simulink model "quad_with_controller"  (R2024b)
settings: configuration reference "prj_default_config" (kept outside this file)
values from neighbouring files (symbols this model uses):
  AngleRope_x = deg2rad(0)    [plant_init.m]
  AngleRope_z = deg2rad(0)    [plant_init.m]
  F_rope = 0    [plant_init.m]
  ModelInit_Att_p = 0    [plant_init.m]
  ModelInit_Att_phi = 0    [plant_init.m]
  ModelInit_Att_psi = 0    [plant_init.m]
  ModelInit_Att_q = 0    [plant_init.m]
  ModelInit_Att_r = 0    [plant_init.m]
  ModelInit_Att_theta = 0    [plant_init.m]
  ModelInit_Pos_Vx = 0    [plant_init.m]
  ModelInit_Pos_Vy = 0    [plant_init.m]
  ModelInit_Pos_Vz = 0    [plant_init.m]
  ModelInit_Pos_x = 0    [plant_init.m]
  ModelInit_Pos_y = 0    [plant_init.m]
  ModelInit_Pos_z = 0    [plant_init.m]
  ModelParam_c_M = 1.489e-07    [plant_init.m]
  ModelParam_c_T = 1.105e-05    [plant_init.m]
  ModelParam_d = 0.225    [plant_init.m]
  ModelParam_g = 9.8    [plant_init.m]
  ModelParam_I_xx = 1.314e-02    (= 0.01314)    [plant_init.m]
  ModelParam_I_yy = 1.314e-02    (= 0.01314)    [plant_init.m]
  ModelParam_I_zz = 2.375e-02    (= 0.02375)    [plant_init.m]
  ModelParam_J_RP = 0.0000986    (= 9.86e-05)    [plant_init.m]
  ModelParam_m = 1.5    [plant_init.m]
libraries: slpidlib x6, mqlib x2
settings Model: Creator=yangyu  LastModifiedBy=yangyu
settings ConfigSetRef: SourceName=prj_default_config  SourceLocation=Base Workspace

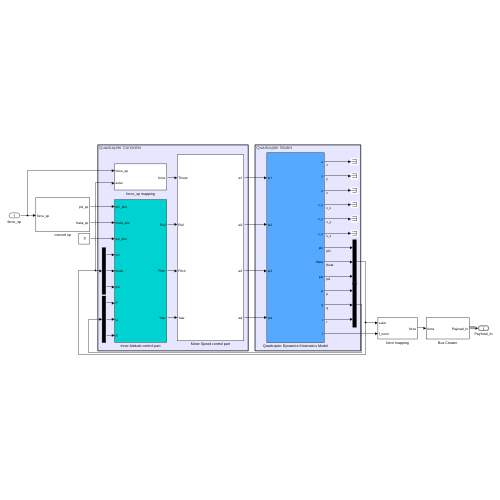
[thumbnail: Simulink's stored preview of the top-level diagram]
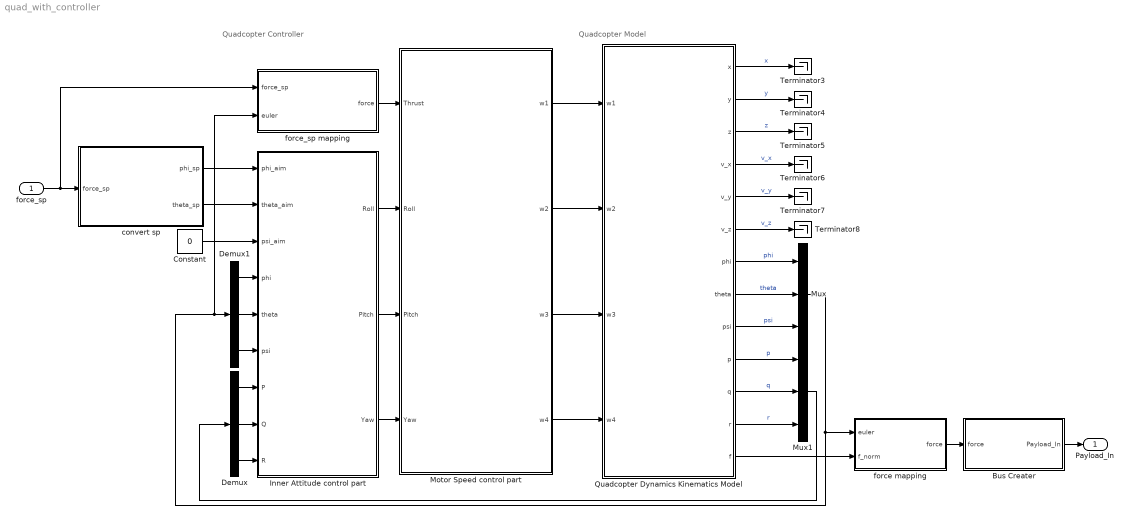
== system quad_with_controller ==
  note: Quadcopter Controller
  note: Quadcopter Model
  force_sp : Inport
  Bus Creater : Subsystem
  Constant : Constant  Value=0
  Demux : Demux  Outputs=3
  Demux1 : Demux  Outputs=3
  Inner Attitude control part : Subsystem
  Motor Speed control part : Subsystem
  Mux : Mux  Inputs=3
  Mux1 : Mux  Inputs=3
  Quadcopter Dynamics Kinematics Model : Subsystem
  Terminator{3..8} (6 alike) : Terminator
  convert sp : Subsystem
  force mapping : Subsystem
  force_sp mapping : Subsystem
  Payload_In : Outport  OutDataTypeStr=Bus: Payload_In_Bus
  wires:
  Motor Speed control part/2(w2) -> Quadcopter Dynamics Kinematics Model/2(w2)
  Motor Speed control part/3(w3) -> Quadcopter Dynamics Kinematics Model/3(w3)
  Motor Speed control part/4(w4) -> Quadcopter Dynamics Kinematics Model/4(w4)
  Quadcopter Dynamics Kinematics Model/10(p) -> Mux1/1  "p"
  Quadcopter Dynamics Kinematics Model/11(q) -> Mux1/2  "q"
  Quadcopter Dynamics Kinematics Model/12(r) -> Mux1/3  "r"
  Quadcopter Dynamics Kinematics Model/1(x) -> Terminator3/1  "x"
  Quadcopter Dynamics Kinematics Model/2(y) -> Terminator4/1  "y"
  Quadcopter Dynamics Kinematics Model/3(z) -> Terminator5/1  "z"
  Quadcopter Dynamics Kinematics Model/4(v_x) -> Terminator6/1  "v_x"
  Quadcopter Dynamics Kinematics Model/5(v_y) -> Terminator7/1  "v_y"
  Quadcopter Dynamics Kinematics Model/6(v_z) -> Terminator8/1  "v_z"
  Quadcopter Dynamics Kinematics Model/7(phi) -> Mux/1  "phi"
  Quadcopter Dynamics Kinematics Model/8(theta) -> Mux/2  "theta"
  Quadcopter Dynamics Kinematics Model/9(psi) -> Mux/3  "psi"
  Bus Creater/1(Payload_In) -> Payload_In/1
  Mux/1 -> force_sp mapping/2(euler), Demux1/1, force mapping/1(euler)
  force mapping/1(force) -> Bus Creater/1(force)
  Inner Attitude control part/3(Yaw) -> Motor Speed control part/4(Yaw)
  Mux1/1 -> Demux/1
  Demux/1 -> Inner Attitude control part/7(P)
  Demux/2 -> Inner Attitude control part/8(Q)
  Demux/3 -> Inner Attitude control part/9(R)
  Demux1/1 -> Inner Attitude control part/4(phi)
  Demux1/2 -> Inner Attitude control part/5(theta)
  Demux1/3 -> Inner Attitude control part/6(psi)
  Constant/1 -> Inner Attitude control part/3(psi_aim)
  force_sp/1 -> force_sp mapping/1(force_sp), convert sp/1(force_sp)
  convert sp/2(theta_sp) -> Inner Attitude control part/2(theta_aim)
  Quadcopter Dynamics Kinematics Model/13(f) -> force mapping/2(f_norm)
  convert sp/1(phi_sp) -> Inner Attitude control part/1(phi_aim)
  Motor Speed control part/1(w1) -> Quadcopter Dynamics Kinematics Model/1(w1)
  force_sp mapping/1(force) -> Motor Speed control part/1(Thrust)
  Inner Attitude control part/1(Roll) -> Motor Speed control part/2(Roll)
  Inner Attitude control part/2(Pitch) -> Motor Speed control part/3(Pitch)

== system quad_with_controller/Bus Creater ==
  force : Inport
  Bus Creator : BusCreator  Inputs=3  OutDataTypeStr=Bus: Payload_In_Bus
  Constant : Constant  Value=zeros(3,1)
  timestamp : mqlib/timestamp
  Payload_In : Outport
  wires:
  force/1 -> Bus Creator/2  "force"
  Bus Creator/1 -> Payload_In/1
  timestamp/1 -> Bus Creator/1  "timestamp"
  Constant/1 -> Bus Creator/3  "moment"

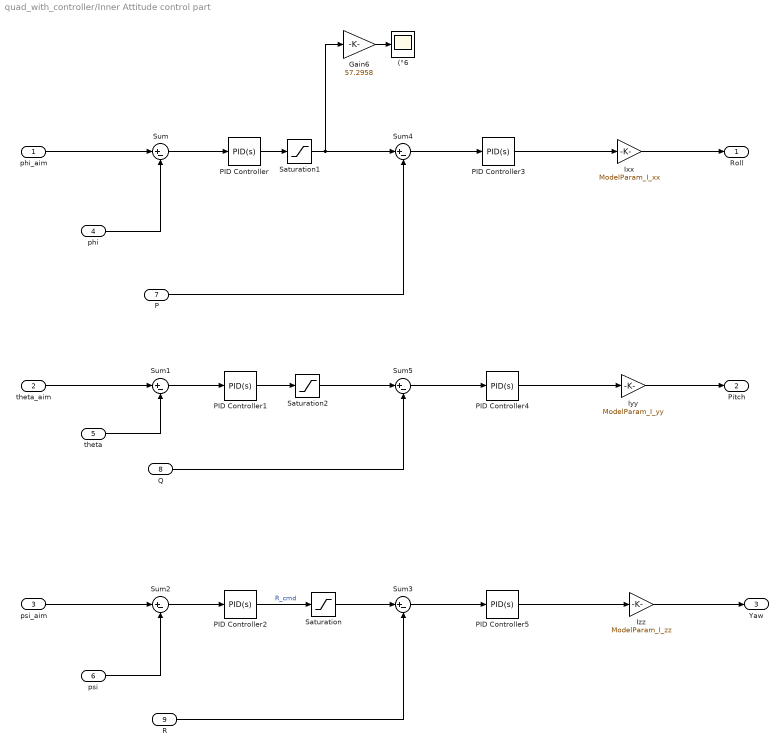
== system quad_with_controller/Inner Attitude control part ==
  phi_aim : Inport
  theta_aim : Inport  Port=2
  psi_aim : Inport  Port=3
  phi : Inport  Port=4
  theta : Inport  Port=5
  psi : Inport  Port=6
  P : Inport  Port=7
  Q : Inport  Port=8
  R : Inport  Port=9
  (°6 : Scope
  Gain6 : Gain  Gain=57.2958
  Ixx : Gain  Gain=ModelParam_I_xx
  Iyy : Gain  Gain=ModelParam_I_yy
  Izz : Gain  Gain=ModelParam_I_zz
  PID Controller : slpidlib/PID Controller  Controller=PID  Form=Parallel  TimeDomain=Continuous-time  UseExternalTs=off  SampleTime=-1  IntegratorMethod=Forward Euler  FilterMethod=Forward Euler  ControllerParametersSource=internal  P=5  I=0  UseKiTs=off  D=0  UseExternalDerivativeSource=off  N=100  UseFilter=on  TunerSelectOption=Transfer Function Based (PID Tuner App)  InitialConditionSource=internal  InitialConditionForIntegrator=0  InitialConditionForFilter=0  DifferentiatorICPrevScaledInput=0  ExternalReset=none  TrackingMode=off  Kt=1  LimitOutput=off  SatLimitsSource=internal  UpperSaturationLimit=inf  LowerSaturationLimit=-inf  LinearizeAsGain=on  AntiWindupMode=none  Kb=1  LimitIntegrator=off  UpperIntegratorSaturationLimit=inf  LowerIntegratorSaturationLimit=-inf  POutMin=[]  POutMax=[]  IOutMin=[]  IOutMax=[]  DOutMin=[]  DOutMax=[]  NOutMin=[]  NOutMax=[]  SumOutMin=[]  SumOutMax=[]  SaturationOutMin=[]  SaturationOutMax=[]  PParamMin=[]  PParamMax=[]  IParamMin=[]  IParamMax=[]  DParamMin=[]  DParamMax=[]  NParamMin=[]  NParamMax=[]  KbParamMin=[]  KbParamMax=[]  KtParamMin=[]  KtParamMax=[]  KbOutMin=[]  KbOutMax=[]  KtOutMin=[]  KtOutMax=[]  IntegratorOutMin=[]  IntegratorOutMax=[]  FilterOutMin=[]  FilterOutMax=[]  SumI1OutMin=[]  SumI1OutMax=[]  SumI2OutMin=[]  SumI2OutMax=[]  SumI3OutMin=[]  SumI3OutMax=[]  SumI4OutMin=[]  SumI4OutMax=[]  SumDOutMin=[]  SumDOutMax=[]  DifferentiatorOutMin=[]  DifferentiatorOutMax=[]  FilterDiffOutCoefMin=[]  FilterDiffOutCoefMax=[]  ReciprocalOutMin=[]  ReciprocalOutMax=[]  SumDenOutMin=[]  SumDenOutMax=[]  SumNumOutMin=[]  SumNumOutMax=[]  DivideOutMin=[]  DivideOutMax=[]  UdiffTsProdOutMin=[]  UdiffTsProdOutMax=[]  NTsProdOutMin=[]  NTsProdOutMax=[]  UintegralTsProdOutMin=[]  UintegralTsProdOutMax=[]  UngainTsProdOutMin=[]  UngainTsProdOutMax=[]  ClampingZeroOutDataTypeStr=Inherit: Inherit via back propagation  ClampingZeroOutMin=[]  ClampingZeroOutMax=[]  FilterDenConstantOutDataTypeStr=Inherit: Inherit via back propagation  FilterDenConstantOutMin=[]  FilterDenConstantOutMax=[]  PCopyOutDataTypeStr=Inherit: Inherit via back propagation  PCopyOutMin=[]  PCopyOutMax=[]  NCopyOutDataTypeStr=Inherit: Inherit via back propagation  NCopyOutMin=[]  NCopyOutMax=[]  IntegratorContinuousStateAttributes=''  IntegratorStateMustResolveToSignalObject=off  IntegratorRTWStateStorageClass=Auto  FilterContinuousStateAttributes=''  FilterStateMustResolveToSignalObject=off  FilterRTWStateStorageClass=Auto  ParallelPVariant=InternalParameters  IdealPVariant=Disabled  IVariant=InternalParameters  DVariant=InternalParameters  IntegratorVariant=Continuous  SatVariant=Disabled  AWVariant=Passthrough  PCopyVariant=Disabled  TRVariant=Disabled  FdbkBlocksVariant=Forward  IdealPFdbkVariant=Disabled  SatFdbkVariant=Disabled  DerivativeFilterVariant=ContFilter  NVariant=InternalParameters  NCopyVariant=Disabled  FilterICVariant=InternalICsFilter  IntegratorICVariant=InternalICs  ExternalResetVariant=Disabled  TRSumVariant=Passthrough  SumFdbkVariant=Disabled  SumVariant=Sum_PID  TsampFilterVariant=InternalTs  TsampNgainVariant=Passthrough  TsampIntegralVariant=Disabled_SignalSpec  ExternalSaturationOutDataTypeStr=Inherit: Same as second input  DerivativeSourceVariant=ErrorSignal  PreIntVariant=InternalPreInt
  PID Controller1 : slpidlib/PID Controller  Controller=PID  Form=Parallel  TimeDomain=Continuous-time  UseExternalTs=off  SampleTime=-1  IntegratorMethod=Forward Euler  FilterMethod=Forward Euler  ControllerParametersSource=internal  P=5  I=0  UseKiTs=off  D=0  UseExternalDerivativeSource=off  N=100  UseFilter=on  TunerSelectOption=Transfer Function Based (PID Tuner App)  InitialConditionSource=internal  InitialConditionForIntegrator=0  InitialConditionForFilter=0  DifferentiatorICPrevScaledInput=0  ExternalReset=none  TrackingMode=off  Kt=1  LimitOutput=off  SatLimitsSource=internal  UpperSaturationLimit=inf  LowerSaturationLimit=-inf  LinearizeAsGain=on  AntiWindupMode=none  Kb=1  LimitIntegrator=off  UpperIntegratorSaturationLimit=inf  LowerIntegratorSaturationLimit=-inf  POutMin=[]  POutMax=[]  IOutMin=[]  IOutMax=[]  DOutMin=[]  DOutMax=[]  NOutMin=[]  NOutMax=[]  SumOutMin=[]  SumOutMax=[]  SaturationOutMin=[]  SaturationOutMax=[]  PParamMin=[]  PParamMax=[]  IParamMin=[]  IParamMax=[]  DParamMin=[]  DParamMax=[]  NParamMin=[]  NParamMax=[]  KbParamMin=[]  KbParamMax=[]  KtParamMin=[]  KtParamMax=[]  KbOutMin=[]  KbOutMax=[]  KtOutMin=[]  KtOutMax=[]  IntegratorOutMin=[]  IntegratorOutMax=[]  FilterOutMin=[]  FilterOutMax=[]  SumI1OutMin=[]  SumI1OutMax=[]  SumI2OutMin=[]  SumI2OutMax=[]  SumI3OutMin=[]  SumI3OutMax=[]  SumI4OutMin=[]  SumI4OutMax=[]  SumDOutMin=[]  SumDOutMax=[]  DifferentiatorOutMin=[]  DifferentiatorOutMax=[]  FilterDiffOutCoefMin=[]  FilterDiffOutCoefMax=[]  ReciprocalOutMin=[]  ReciprocalOutMax=[]  SumDenOutMin=[]  SumDenOutMax=[]  SumNumOutMin=[]  SumNumOutMax=[]  DivideOutMin=[]  DivideOutMax=[]  UdiffTsProdOutMin=[]  UdiffTsProdOutMax=[]  NTsProdOutMin=[]  NTsProdOutMax=[]  UintegralTsProdOutMin=[]  UintegralTsProdOutMax=[]  UngainTsProdOutMin=[]  UngainTsProdOutMax=[]  ClampingZeroOutDataTypeStr=Inherit: Inherit via back propagation  ClampingZeroOutMin=[]  ClampingZeroOutMax=[]  FilterDenConstantOutDataTypeStr=Inherit: Inherit via back propagation  FilterDenConstantOutMin=[]  FilterDenConstantOutMax=[]  PCopyOutDataTypeStr=Inherit: Inherit via back propagation  PCopyOutMin=[]  PCopyOutMax=[]  NCopyOutDataTypeStr=Inherit: Inherit via back propagation  NCopyOutMin=[]  NCopyOutMax=[]  IntegratorContinuousStateAttributes=''  IntegratorStateMustResolveToSignalObject=off  IntegratorRTWStateStorageClass=Auto  FilterContinuousStateAttributes=''  FilterStateMustResolveToSignalObject=off  FilterRTWStateStorageClass=Auto  ParallelPVariant=InternalParameters  IdealPVariant=Disabled  IVariant=InternalParameters  DVariant=InternalParameters  IntegratorVariant=Continuous  SatVariant=Disabled  AWVariant=Passthrough  PCopyVariant=Disabled  TRVariant=Disabled  FdbkBlocksVariant=Forward  IdealPFdbkVariant=Disabled  SatFdbkVariant=Disabled  DerivativeFilterVariant=ContFilter  NVariant=InternalParameters  NCopyVariant=Disabled  FilterICVariant=InternalICsFilter  IntegratorICVariant=InternalICs  ExternalResetVariant=Disabled  TRSumVariant=Passthrough  SumFdbkVariant=Disabled  SumVariant=Sum_PID  TsampFilterVariant=InternalTs  TsampNgainVariant=Passthrough  TsampIntegralVariant=Disabled_SignalSpec  ExternalSaturationOutDataTypeStr=Inherit: Same as second input  DerivativeSourceVariant=ErrorSignal  PreIntVariant=InternalPreInt
  PID Controller2 : slpidlib/PID Controller  Controller=PID  Form=Parallel  TimeDomain=Continuous-time  UseExternalTs=off  SampleTime=-1  IntegratorMethod=Forward Euler  FilterMethod=Forward Euler  ControllerParametersSource=internal  P=5  I=0  UseKiTs=off  D=0  UseExternalDerivativeSource=off  N=1000  UseFilter=on  TunerSelectOption=Transfer Function Based (PID Tuner App)  InitialConditionSource=internal  InitialConditionForIntegrator=0  InitialConditionForFilter=0  DifferentiatorICPrevScaledInput=0  ExternalReset=none  TrackingMode=off  Kt=1  LimitOutput=off  SatLimitsSource=internal  UpperSaturationLimit=inf  LowerSaturationLimit=-inf  LinearizeAsGain=on  AntiWindupMode=none  Kb=1  LimitIntegrator=off  UpperIntegratorSaturationLimit=inf  LowerIntegratorSaturationLimit=-inf  POutMin=[]  POutMax=[]  IOutMin=[]  IOutMax=[]  DOutMin=[]  DOutMax=[]  NOutMin=[]  NOutMax=[]  SumOutMin=[]  SumOutMax=[]  SaturationOutMin=[]  SaturationOutMax=[]  PParamMin=[]  PParamMax=[]  IParamMin=[]  IParamMax=[]  DParamMin=[]  DParamMax=[]  NParamMin=[]  NParamMax=[]  KbParamMin=[]  KbParamMax=[]  KtParamMin=[]  KtParamMax=[]  KbOutMin=[]  KbOutMax=[]  KtOutMin=[]  KtOutMax=[]  IntegratorOutMin=[]  IntegratorOutMax=[]  FilterOutMin=[]  FilterOutMax=[]  SumI1OutMin=[]  SumI1OutMax=[]  SumI2OutMin=[]  SumI2OutMax=[]  SumI3OutMin=[]  SumI3OutMax=[]  SumI4OutMin=[]  SumI4OutMax=[]  SumDOutMin=[]  SumDOutMax=[]  DifferentiatorOutMin=[]  DifferentiatorOutMax=[]  FilterDiffOutCoefMin=[]  FilterDiffOutCoefMax=[]  ReciprocalOutMin=[]  ReciprocalOutMax=[]  SumDenOutMin=[]  SumDenOutMax=[]  SumNumOutMin=[]  SumNumOutMax=[]  DivideOutMin=[]  DivideOutMax=[]  UdiffTsProdOutMin=[]  UdiffTsProdOutMax=[]  NTsProdOutMin=[]  NTsProdOutMax=[]  UintegralTsProdOutMin=[]  UintegralTsProdOutMax=[]  UngainTsProdOutMin=[]  UngainTsProdOutMax=[]  ClampingZeroOutDataTypeStr=Inherit: Inherit via back propagation  ClampingZeroOutMin=[]  ClampingZeroOutMax=[]  FilterDenConstantOutDataTypeStr=Inherit: Inherit via back propagation  FilterDenConstantOutMin=[]  FilterDenConstantOutMax=[]  PCopyOutDataTypeStr=Inherit: Inherit via back propagation  PCopyOutMin=[]  PCopyOutMax=[]  NCopyOutDataTypeStr=Inherit: Inherit via back propagation  NCopyOutMin=[]  NCopyOutMax=[]  IntegratorContinuousStateAttributes=''  IntegratorStateMustResolveToSignalObject=off  IntegratorRTWStateStorageClass=Auto  FilterContinuousStateAttributes=''  FilterStateMustResolveToSignalObject=off  FilterRTWStateStorageClass=Auto  ParallelPVariant=InternalParameters  IdealPVariant=Disabled  IVariant=InternalParameters  DVariant=InternalParameters  IntegratorVariant=Continuous  SatVariant=Disabled  AWVariant=Passthrough  PCopyVariant=Disabled  TRVariant=Disabled  FdbkBlocksVariant=Forward  IdealPFdbkVariant=Disabled  SatFdbkVariant=Disabled  DerivativeFilterVariant=ContFilter  NVariant=InternalParameters  NCopyVariant=Disabled  FilterICVariant=InternalICsFilter  IntegratorICVariant=InternalICs  ExternalResetVariant=Disabled  TRSumVariant=Passthrough  SumFdbkVariant=Disabled  SumVariant=Sum_PID  TsampFilterVariant=InternalTs  TsampNgainVariant=Passthrough  TsampIntegralVariant=Disabled_SignalSpec  ExternalSaturationOutDataTypeStr=Inherit: Same as second input  DerivativeSourceVariant=ErrorSignal  PreIntVariant=InternalPreInt
  PID Controller3 : slpidlib/PID Controller  Controller=PID  Form=Parallel  TimeDomain=Continuous-time  UseExternalTs=off  SampleTime=-1  IntegratorMethod=Forward Euler  FilterMethod=Forward Euler  ControllerParametersSource=internal  P=15  I=0  UseKiTs=off  D=0  UseExternalDerivativeSource=off  N=1000  UseFilter=on  TunerSelectOption=Transfer Function Based (PID Tuner App)  InitialConditionSource=internal  InitialConditionForIntegrator=0  InitialConditionForFilter=0  DifferentiatorICPrevScaledInput=0  ExternalReset=none  TrackingMode=off  Kt=1  LimitOutput=off  SatLimitsSource=internal  UpperSaturationLimit=inf  LowerSaturationLimit=-inf  LinearizeAsGain=on  AntiWindupMode=none  Kb=1  LimitIntegrator=off  UpperIntegratorSaturationLimit=inf  LowerIntegratorSaturationLimit=-inf  POutMin=[]  POutMax=[]  IOutMin=[]  IOutMax=[]  DOutMin=[]  DOutMax=[]  NOutMin=[]  NOutMax=[]  SumOutMin=[]  SumOutMax=[]  SaturationOutMin=[]  SaturationOutMax=[]  PParamMin=[]  PParamMax=[]  IParamMin=[]  IParamMax=[]  DParamMin=[]  DParamMax=[]  NParamMin=[]  NParamMax=[]  KbParamMin=[]  KbParamMax=[]  KtParamMin=[]  KtParamMax=[]  KbOutMin=[]  KbOutMax=[]  KtOutMin=[]  KtOutMax=[]  IntegratorOutMin=[]  IntegratorOutMax=[]  FilterOutMin=[]  FilterOutMax=[]  SumI1OutMin=[]  SumI1OutMax=[]  SumI2OutMin=[]  SumI2OutMax=[]  SumI3OutMin=[]  SumI3OutMax=[]  SumI4OutMin=[]  SumI4OutMax=[]  SumDOutMin=[]  SumDOutMax=[]  DifferentiatorOutMin=[]  DifferentiatorOutMax=[]  FilterDiffOutCoefMin=[]  FilterDiffOutCoefMax=[]  ReciprocalOutMin=[]  ReciprocalOutMax=[]  SumDenOutMin=[]  SumDenOutMax=[]  SumNumOutMin=[]  SumNumOutMax=[]  DivideOutMin=[]  DivideOutMax=[]  UdiffTsProdOutMin=[]  UdiffTsProdOutMax=[]  NTsProdOutMin=[]  NTsProdOutMax=[]  UintegralTsProdOutMin=[]  UintegralTsProdOutMax=[]  UngainTsProdOutMin=[]  UngainTsProdOutMax=[]  ClampingZeroOutDataTypeStr=Inherit: Inherit via back propagation  ClampingZeroOutMin=[]  ClampingZeroOutMax=[]  FilterDenConstantOutDataTypeStr=Inherit: Inherit via back propagation  FilterDenConstantOutMin=[]  FilterDenConstantOutMax=[]  PCopyOutDataTypeStr=Inherit: Inherit via back propagation  PCopyOutMin=[]  PCopyOutMax=[]  NCopyOutDataTypeStr=Inherit: Inherit via back propagation  NCopyOutMin=[]  NCopyOutMax=[]  IntegratorContinuousStateAttributes=''  IntegratorStateMustResolveToSignalObject=off  IntegratorRTWStateStorageClass=Auto  FilterContinuousStateAttributes=''  FilterStateMustResolveToSignalObject=off  FilterRTWStateStorageClass=Auto  ParallelPVariant=InternalParameters  IdealPVariant=Disabled  IVariant=InternalParameters  DVariant=InternalParameters  IntegratorVariant=Continuous  SatVariant=Disabled  AWVariant=Passthrough  PCopyVariant=Disabled  TRVariant=Disabled  FdbkBlocksVariant=Forward  IdealPFdbkVariant=Disabled  SatFdbkVariant=Disabled  DerivativeFilterVariant=ContFilter  NVariant=InternalParameters  NCopyVariant=Disabled  FilterICVariant=InternalICsFilter  IntegratorICVariant=InternalICs  ExternalResetVariant=Disabled  TRSumVariant=Passthrough  SumFdbkVariant=Disabled  SumVariant=Sum_PID  TsampFilterVariant=InternalTs  TsampNgainVariant=Passthrough  TsampIntegralVariant=Disabled_SignalSpec  ExternalSaturationOutDataTypeStr=Inherit: Same as second input  DerivativeSourceVariant=ErrorSignal  PreIntVariant=InternalPreInt
  PID Controller4 : slpidlib/PID Controller  Controller=PID  Form=Parallel  TimeDomain=Continuous-time  UseExternalTs=off  SampleTime=-1  IntegratorMethod=Forward Euler  FilterMethod=Forward Euler  ControllerParametersSource=internal  P=15  I=0  UseKiTs=off  D=0  UseExternalDerivativeSource=off  N=1000  UseFilter=on  TunerSelectOption=Transfer Function Based (PID Tuner App)  InitialConditionSource=internal  InitialConditionForIntegrator=0  InitialConditionForFilter=0  DifferentiatorICPrevScaledInput=0  ExternalReset=none  TrackingMode=off  Kt=1  LimitOutput=off  SatLimitsSource=internal  UpperSaturationLimit=inf  LowerSaturationLimit=-inf  LinearizeAsGain=on  AntiWindupMode=none  Kb=1  LimitIntegrator=off  UpperIntegratorSaturationLimit=inf  LowerIntegratorSaturationLimit=-inf  POutMin=[]  POutMax=[]  IOutMin=[]  IOutMax=[]  DOutMin=[]  DOutMax=[]  NOutMin=[]  NOutMax=[]  SumOutMin=[]  SumOutMax=[]  SaturationOutMin=[]  SaturationOutMax=[]  PParamMin=[]  PParamMax=[]  IParamMin=[]  IParamMax=[]  DParamMin=[]  DParamMax=[]  NParamMin=[]  NParamMax=[]  KbParamMin=[]  KbParamMax=[]  KtParamMin=[]  KtParamMax=[]  KbOutMin=[]  KbOutMax=[]  KtOutMin=[]  KtOutMax=[]  IntegratorOutMin=[]  IntegratorOutMax=[]  FilterOutMin=[]  FilterOutMax=[]  SumI1OutMin=[]  SumI1OutMax=[]  SumI2OutMin=[]  SumI2OutMax=[]  SumI3OutMin=[]  SumI3OutMax=[]  SumI4OutMin=[]  SumI4OutMax=[]  SumDOutMin=[]  SumDOutMax=[]  DifferentiatorOutMin=[]  DifferentiatorOutMax=[]  FilterDiffOutCoefMin=[]  FilterDiffOutCoefMax=[]  ReciprocalOutMin=[]  ReciprocalOutMax=[]  SumDenOutMin=[]  SumDenOutMax=[]  SumNumOutMin=[]  SumNumOutMax=[]  DivideOutMin=[]  DivideOutMax=[]  UdiffTsProdOutMin=[]  UdiffTsProdOutMax=[]  NTsProdOutMin=[]  NTsProdOutMax=[]  UintegralTsProdOutMin=[]  UintegralTsProdOutMax=[]  UngainTsProdOutMin=[]  UngainTsProdOutMax=[]  ClampingZeroOutDataTypeStr=Inherit: Inherit via back propagation  ClampingZeroOutMin=[]  ClampingZeroOutMax=[]  FilterDenConstantOutDataTypeStr=Inherit: Inherit via back propagation  FilterDenConstantOutMin=[]  FilterDenConstantOutMax=[]  PCopyOutDataTypeStr=Inherit: Inherit via back propagation  PCopyOutMin=[]  PCopyOutMax=[]  NCopyOutDataTypeStr=Inherit: Inherit via back propagation  NCopyOutMin=[]  NCopyOutMax=[]  IntegratorContinuousStateAttributes=''  IntegratorStateMustResolveToSignalObject=off  IntegratorRTWStateStorageClass=Auto  FilterContinuousStateAttributes=''  FilterStateMustResolveToSignalObject=off  FilterRTWStateStorageClass=Auto  ParallelPVariant=InternalParameters  IdealPVariant=Disabled  IVariant=InternalParameters  DVariant=InternalParameters  IntegratorVariant=Continuous  SatVariant=Disabled  AWVariant=Passthrough  PCopyVariant=Disabled  TRVariant=Disabled  FdbkBlocksVariant=Forward  IdealPFdbkVariant=Disabled  SatFdbkVariant=Disabled  DerivativeFilterVariant=ContFilter  NVariant=InternalParameters  NCopyVariant=Disabled  FilterICVariant=InternalICsFilter  IntegratorICVariant=InternalICs  ExternalResetVariant=Disabled  TRSumVariant=Passthrough  SumFdbkVariant=Disabled  SumVariant=Sum_PID  TsampFilterVariant=InternalTs  TsampNgainVariant=Passthrough  TsampIntegralVariant=Disabled_SignalSpec  ExternalSaturationOutDataTypeStr=Inherit: Same as second input  DerivativeSourceVariant=ErrorSignal  PreIntVariant=InternalPreInt
  PID Controller5 : slpidlib/PID Controller  Controller=PID  Form=Parallel  TimeDomain=Continuous-time  UseExternalTs=off  SampleTime=-1  IntegratorMethod=Forward Euler  FilterMethod=Forward Euler  ControllerParametersSource=internal  P=15  I=0  UseKiTs=off  D=0  UseExternalDerivativeSource=off  N=1000  UseFilter=on  TunerSelectOption=Transfer Function Based (PID Tuner App)  InitialConditionSource=internal  InitialConditionForIntegrator=0  InitialConditionForFilter=0  DifferentiatorICPrevScaledInput=0  ExternalReset=none  TrackingMode=off  Kt=1  LimitOutput=off  SatLimitsSource=internal  UpperSaturationLimit=inf  LowerSaturationLimit=-inf  LinearizeAsGain=on  AntiWindupMode=none  Kb=1  LimitIntegrator=off  UpperIntegratorSaturationLimit=inf  LowerIntegratorSaturationLimit=-inf  POutMin=[]  POutMax=[]  IOutMin=[]  IOutMax=[]  DOutMin=[]  DOutMax=[]  NOutMin=[]  NOutMax=[]  SumOutMin=[]  SumOutMax=[]  SaturationOutMin=[]  SaturationOutMax=[]  PParamMin=[]  PParamMax=[]  IParamMin=[]  IParamMax=[]  DParamMin=[]  DParamMax=[]  NParamMin=[]  NParamMax=[]  KbParamMin=[]  KbParamMax=[]  KtParamMin=[]  KtParamMax=[]  KbOutMin=[]  KbOutMax=[]  KtOutMin=[]  KtOutMax=[]  IntegratorOutMin=[]  IntegratorOutMax=[]  FilterOutMin=[]  FilterOutMax=[]  SumI1OutMin=[]  SumI1OutMax=[]  SumI2OutMin=[]  SumI2OutMax=[]  SumI3OutMin=[]  SumI3OutMax=[]  SumI4OutMin=[]  SumI4OutMax=[]  SumDOutMin=[]  SumDOutMax=[]  DifferentiatorOutMin=[]  DifferentiatorOutMax=[]  FilterDiffOutCoefMin=[]  FilterDiffOutCoefMax=[]  ReciprocalOutMin=[]  ReciprocalOutMax=[]  SumDenOutMin=[]  SumDenOutMax=[]  SumNumOutMin=[]  SumNumOutMax=[]  DivideOutMin=[]  DivideOutMax=[]  UdiffTsProdOutMin=[]  UdiffTsProdOutMax=[]  NTsProdOutMin=[]  NTsProdOutMax=[]  UintegralTsProdOutMin=[]  UintegralTsProdOutMax=[]  UngainTsProdOutMin=[]  UngainTsProdOutMax=[]  ClampingZeroOutDataTypeStr=Inherit: Inherit via back propagation  ClampingZeroOutMin=[]  ClampingZeroOutMax=[]  FilterDenConstantOutDataTypeStr=Inherit: Inherit via back propagation  FilterDenConstantOutMin=[]  FilterDenConstantOutMax=[]  PCopyOutDataTypeStr=Inherit: Inherit via back propagation  PCopyOutMin=[]  PCopyOutMax=[]  NCopyOutDataTypeStr=Inherit: Inherit via back propagation  NCopyOutMin=[]  NCopyOutMax=[]  IntegratorContinuousStateAttributes=''  IntegratorStateMustResolveToSignalObject=off  IntegratorRTWStateStorageClass=Auto  FilterContinuousStateAttributes=''  FilterStateMustResolveToSignalObject=off  FilterRTWStateStorageClass=Auto  ParallelPVariant=InternalParameters  IdealPVariant=Disabled  IVariant=InternalParameters  DVariant=InternalParameters  IntegratorVariant=Continuous  SatVariant=Disabled  AWVariant=Passthrough  PCopyVariant=Disabled  TRVariant=Disabled  FdbkBlocksVariant=Forward  IdealPFdbkVariant=Disabled  SatFdbkVariant=Disabled  DerivativeFilterVariant=ContFilter  NVariant=InternalParameters  NCopyVariant=Disabled  FilterICVariant=InternalICsFilter  IntegratorICVariant=InternalICs  ExternalResetVariant=Disabled  TRSumVariant=Passthrough  SumFdbkVariant=Disabled  SumVariant=Sum_PID  TsampFilterVariant=InternalTs  TsampNgainVariant=Passthrough  TsampIntegralVariant=Disabled_SignalSpec  ExternalSaturationOutDataTypeStr=Inherit: Same as second input  DerivativeSourceVariant=ErrorSignal  PreIntVariant=InternalPreInt
  Saturation : Saturate  UpperLimit=deg2rad(90)  LowerLimit=-deg2rad(90)
  Saturation1 : Saturate  UpperLimit=deg2rad(180)  LowerLimit=-deg2rad(180)
  Saturation2 : Saturate  UpperLimit=deg2rad(180)  LowerLimit=-deg2rad(180)
  Sum{,1..5} (6 alike) : Sum  Inputs=|+-
  Roll : Outport
  Pitch : Outport  Port=2
  Yaw : Outport  Port=3
  wires:
  psi_aim/1 -> Sum2/1
  Ixx/1 -> Roll/1
  Sum2/1 -> PID Controller2/1
  Sum1/1 -> PID Controller1/1
  Izz/1 -> Yaw/1
  phi/1 -> Sum/2
  phi_aim/1 -> Sum/1
  Iyy/1 -> Pitch/1
  psi/1 -> Sum2/2
  theta/1 -> Sum1/2
  theta_aim/1 -> Sum1/1
  PID Controller2/1 -> Saturation/1  "R_cmd"
  Sum3/1 -> PID Controller5/1
  PID Controller1/1 -> Saturation2/1
  Sum5/1 -> PID Controller4/1
  Q/1 -> Sum5/2
  PID Controller4/1 -> Iyy/1
  P/1 -> Sum4/2
  R/1 -> Sum3/2
  PID Controller5/1 -> Izz/1
  Saturation/1 -> Sum3/1
  Sum4/1 -> PID Controller3/1
  Sum/1 -> PID Controller/1
  Gain6/1 -> (°6/1
  PID Controller3/1 -> Ixx/1
  PID Controller/1 -> Saturation1/1
  Saturation1/1 -> Gain6/1, Sum4/1
  Saturation2/1 -> Sum5/1

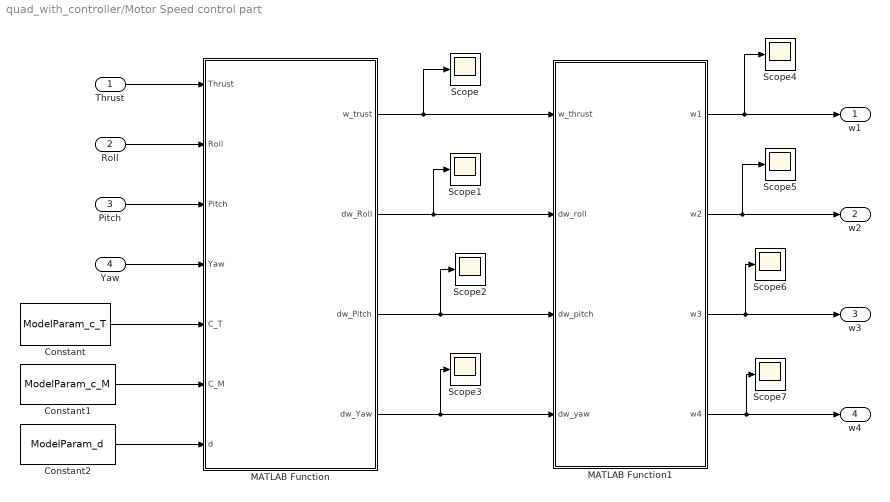
== system quad_with_controller/Motor Speed control part ==
  Thrust : Inport
  Roll : Inport  Port=2
  Pitch : Inport  Port=3
  Yaw : Inport  Port=4
  Constant : Constant  Value=ModelParam_c_T
  Constant1 : Constant  Value=ModelParam_c_M
  Constant2 : Constant  Value=ModelParam_d
  MATLAB Function : MATLAB Function  TreatAsAtomicUnit=on
  MATLAB Function1 : MATLAB Function  TreatAsAtomicUnit=on
  Scope{,1..7} (8 alike) : Scope
  w1 : Outport
  w2 : Outport  Port=2
  w3 : Outport  Port=3
  w4 : Outport  Port=4
  wires:
  MATLAB Function/3(dw_Pitch) -> Scope2/1, MATLAB Function1/3(dw_pitch)
  Thrust/1 -> MATLAB Function/1(Thrust)
  Roll/1 -> MATLAB Function/2(Roll)
  Pitch/1 -> MATLAB Function/3(Pitch)
  Yaw/1 -> MATLAB Function/4(Yaw)
  Constant/1 -> MATLAB Function/5(C_T)
  Constant1/1 -> MATLAB Function/6(C_M)
  Constant2/1 -> MATLAB Function/7(d)
  MATLAB Function1/1(w1) -> w1/1, Scope4/1
  MATLAB Function1/2(w2) -> w2/1, Scope5/1
  MATLAB Function1/3(w3) -> w3/1, Scope6/1
  MATLAB Function1/4(w4) -> w4/1, Scope7/1
  MATLAB Function/4(dw_Yaw) -> Scope3/1, MATLAB Function1/4(dw_yaw)
  MATLAB Function/1(w_trust) -> Scope/1, MATLAB Function1/1(w_thrust)
  MATLAB Function/2(dw_Roll) -> Scope1/1, MATLAB Function1/2(dw_roll)

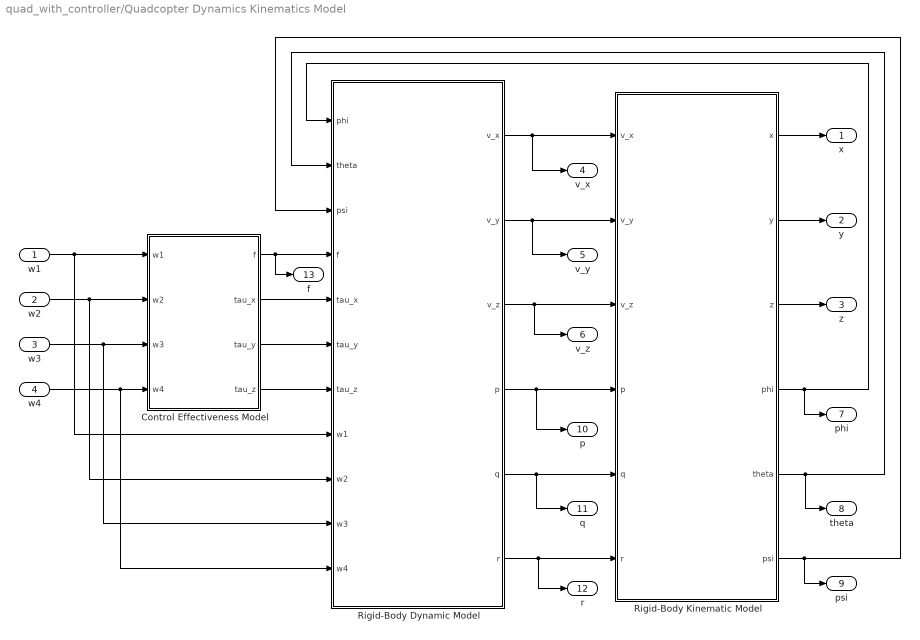
== system quad_with_controller/Quadcopter Dynamics Kinematics Model ==
  w1 : Inport
  w2 : Inport  Port=2
  w3 : Inport  Port=3
  w4 : Inport  Port=4
  Control Effectiveness Model : Subsystem
  Rigid-Body Dynamic Model : Subsystem
  Rigid-Body Kinematic Model : Subsystem
  x : Outport  VectorParamsAs1DForOutWhenUnconnected=off
  y : Outport  Port=2  VectorParamsAs1DForOutWhenUnconnected=off
  z : Outport  Port=3  VectorParamsAs1DForOutWhenUnconnected=off
  v_x : Outport  Port=4  VectorParamsAs1DForOutWhenUnconnected=off
  v_y : Outport  Port=5  VectorParamsAs1DForOutWhenUnconnected=off
  v_z : Outport  Port=6  VectorParamsAs1DForOutWhenUnconnected=off
  phi : Outport  Port=7  VectorParamsAs1DForOutWhenUnconnected=off
  theta : Outport  Port=8  VectorParamsAs1DForOutWhenUnconnected=off
  psi : Outport  Port=9  VectorParamsAs1DForOutWhenUnconnected=off
  p : Outport  Port=10  VectorParamsAs1DForOutWhenUnconnected=off
  q : Outport  Port=11  VectorParamsAs1DForOutWhenUnconnected=off
  r : Outport  Port=12  VectorParamsAs1DForOutWhenUnconnected=off
  f : Outport  Port=13
  wires:
  w1/1 -> Rigid-Body Dynamic Model/8(w1), Control Effectiveness Model/1(w1)
  Control Effectiveness Model/1(f) -> f/1, Rigid-Body Dynamic Model/4(f)
  w3/1 -> Rigid-Body Dynamic Model/10(w3), Control Effectiveness Model/3(w3)
  Rigid-Body Kinematic Model/5(theta) -> theta/1, Rigid-Body Dynamic Model/2(theta)
  w4/1 -> Rigid-Body Dynamic Model/11(w4), Control Effectiveness Model/4(w4)
  Rigid-Body Kinematic Model/4(phi) -> Rigid-Body Dynamic Model/1(phi), phi/1
  w2/1 -> Rigid-Body Dynamic Model/9(w2), Control Effectiveness Model/2(w2)
  Rigid-Body Dynamic Model/4(p) -> Rigid-Body Kinematic Model/4(p), p/1
  Rigid-Body Dynamic Model/3(v_z) -> Rigid-Body Kinematic Model/3(v_z), v_z/1
  Rigid-Body Dynamic Model/6(r) -> Rigid-Body Kinematic Model/6(r), r/1
  Control Effectiveness Model/2(tau_x) -> Rigid-Body Dynamic Model/5(tau_x)
  Rigid-Body Dynamic Model/2(v_y) -> Rigid-Body Kinematic Model/2(v_y), v_y/1
  Rigid-Body Kinematic Model/1(x) -> x/1
  Rigid-Body Kinematic Model/6(psi) -> psi/1, Rigid-Body Dynamic Model/3(psi)
  Rigid-Body Dynamic Model/5(q) -> Rigid-Body Kinematic Model/5(q), q/1
  Control Effectiveness Model/4(tau_z) -> Rigid-Body Dynamic Model/7(tau_z)
  Rigid-Body Kinematic Model/2(y) -> y/1
  Rigid-Body Kinematic Model/3(z) -> z/1
  Rigid-Body Dynamic Model/1(v_x) -> v_x/1, Rigid-Body Kinematic Model/1(v_x)
  Control Effectiveness Model/3(tau_y) -> Rigid-Body Dynamic Model/6(tau_y)

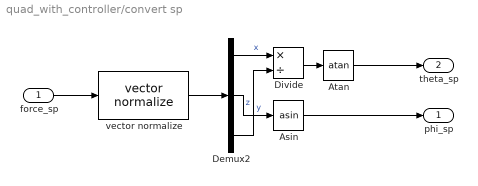
== system quad_with_controller/convert sp ==
  force_sp : Inport
  Asin : Trigonometry  Operator=asin
  Atan : Trigonometry  Operator=atan
  Demux2 : Demux  Outputs=3
  Divide : Product  Inputs=*/
  vector normalize : mqlib/vector normalize
  phi_sp : Outport
  theta_sp : Outport  Port=2
  wires:
  Demux2/2 -> Asin/1  "y"
  Demux2/1 -> Divide/1  "x"
  force_sp/1 -> vector normalize/1
  Demux2/3 -> Divide/2  "z"
  Divide/1 -> Atan/1
  vector normalize/1 -> Demux2/1
  Atan/1 -> theta_sp/1
  Asin/1 -> phi_sp/1

== system quad_with_controller/force mapping ==
  euler : Inport
  f_norm : Inport  Port=2
  Constant : Constant  Value=[0;0;-1]
  Euler To DCM : Subsystem
  Matrix Multiply : Product  Multiplication=Matrix(*)
  Product : Product
  force : Outport
  wires:
  Constant/1 -> Matrix Multiply/2
  Euler To DCM/1(R) -> Matrix Multiply/1
  f_norm/1 -> Product/2
  euler/1 -> Euler To DCM/1(euler)
  Matrix Multiply/1 -> Product/1
  Product/1 -> force/1

== system quad_with_controller/force_sp mapping ==
  force_sp : Inport
  euler : Inport  Port=2
  Constant1 : Constant  Value=[0;0;-1]
  Dot Product : DotProduct  OutDataTypeStr=Inherit: Inherit via internal rule
  Euler To DCM : Subsystem
  Matrix Multiply : Product  Multiplication=Matrix(*)
  force : Outport
  wires:
  Constant1/1 -> Matrix Multiply/2
  Matrix Multiply/1 -> Dot Product/1
  Dot Product/1 -> force/1
  Euler To DCM/1(R) -> Matrix Multiply/1
  euler/1 -> Euler To DCM/1(euler)
  force_sp/1 -> Dot Product/2

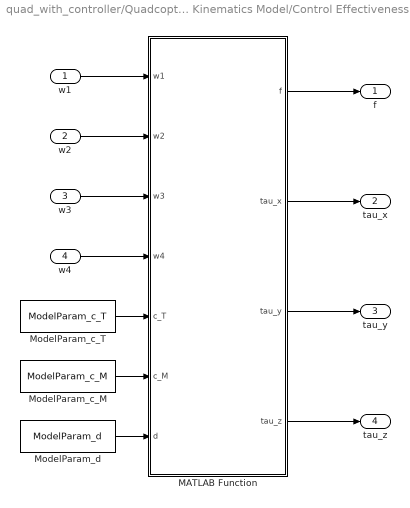
== system quad_with_controller/Quadcopter Dynamics Kinematics Model/Control Effectiveness Model ==
  w1 : Inport
  w2 : Inport  Port=2
  w3 : Inport  Port=3
  w4 : Inport  Port=4
  MATLAB Function : MATLAB Function  TreatAsAtomicUnit=on
  ModelParam_c_M : Constant  Value=ModelParam_c_M
  ModelParam_c_T : Constant  Value=ModelParam_c_T
  ModelParam_d : Constant  Value=ModelParam_d
  f : Outport  VectorParamsAs1DForOutWhenUnconnected=off
  tau_x : Outport  Port=2  VectorParamsAs1DForOutWhenUnconnected=off
  tau_y : Outport  Port=3  VectorParamsAs1DForOutWhenUnconnected=off
  tau_z : Outport  Port=4  VectorParamsAs1DForOutWhenUnconnected=off
  wires:
  ModelParam_c_M/1 -> MATLAB Function/6(c_M)
  ModelParam_c_T/1 -> MATLAB Function/5(c_T)
  MATLAB Function/3(tau_y) -> tau_y/1
  MATLAB Function/1(f) -> f/1
  ModelParam_d/1 -> MATLAB Function/7(d)
  MATLAB Function/4(tau_z) -> tau_z/1
  w3/1 -> MATLAB Function/3(w3)
  w1/1 -> MATLAB Function/1(w1)
  w4/1 -> MATLAB Function/4(w4)
  MATLAB Function/2(tau_x) -> tau_x/1
  w2/1 -> MATLAB Function/2(w2)

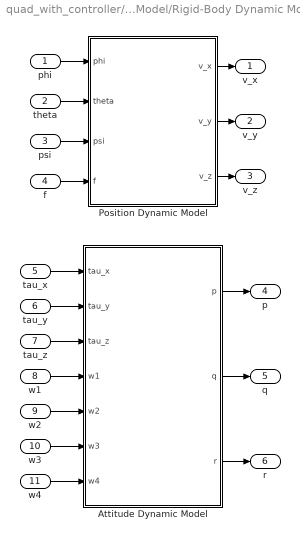
== system quad_with_controller/Quadcopter Dynamics Kinematics Model/Rigid-Body Dynamic Model ==
  phi : Inport
  theta : Inport  Port=2
  psi : Inport  Port=3
  f : Inport  Port=4
  tau_x : Inport  Port=5
  tau_y : Inport  Port=6
  tau_z : Inport  Port=7
  w1 : Inport  Port=8
  w2 : Inport  Port=9
  w3 : Inport  Port=10
  w4 : Inport  Port=11
  Attitude Dynamic Model : Subsystem
  Position Dynamic Model : Subsystem
  v_x : Outport  VectorParamsAs1DForOutWhenUnconnected=off
  v_y : Outport  Port=2  VectorParamsAs1DForOutWhenUnconnected=off
  v_z : Outport  Port=3  VectorParamsAs1DForOutWhenUnconnected=off
  p : Outport  Port=4  VectorParamsAs1DForOutWhenUnconnected=off
  q : Outport  Port=5  VectorParamsAs1DForOutWhenUnconnected=off
  r : Outport  Port=6  VectorParamsAs1DForOutWhenUnconnected=off
  wires:
  w3/1 -> Attitude Dynamic Model/6(w3)
  w1/1 -> Attitude Dynamic Model/4(w1)
  theta/1 -> Position Dynamic Model/2(theta)
  f/1 -> Position Dynamic Model/4(f)
  tau_x/1 -> Attitude Dynamic Model/1(tau_x)
  w2/1 -> Attitude Dynamic Model/5(w2)
  Attitude Dynamic Model/1(p) -> p/1
  w4/1 -> Attitude Dynamic Model/7(w4)
  Attitude Dynamic Model/2(q) -> q/1
  tau_y/1 -> Attitude Dynamic Model/2(tau_y)
  tau_z/1 -> Attitude Dynamic Model/3(tau_z)
  Position Dynamic Model/3(v_z) -> v_z/1
  Attitude Dynamic Model/3(r) -> r/1
  phi/1 -> Position Dynamic Model/1(phi)
  psi/1 -> Position Dynamic Model/3(psi)
  Position Dynamic Model/1(v_x) -> v_x/1
  Position Dynamic Model/2(v_y) -> v_y/1

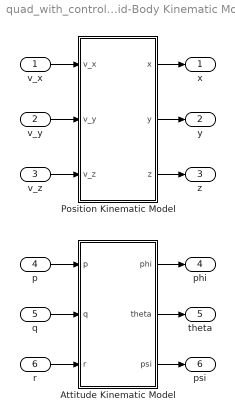
== system quad_with_controller/Quadcopter Dynamics Kinematics Model/Rigid-Body Kinematic Model ==
  v_x : Inport
  v_y : Inport  Port=2
  v_z : Inport  Port=3
  p : Inport  Port=4
  q : Inport  Port=5
  r : Inport  Port=6
  Attitude Kinematic Model : Subsystem
  Position Kinematic Model : Subsystem
  x : Outport  VectorParamsAs1DForOutWhenUnconnected=off
  y : Outport  Port=2  VectorParamsAs1DForOutWhenUnconnected=off
  z : Outport  Port=3  VectorParamsAs1DForOutWhenUnconnected=off
  phi : Outport  Port=4  VectorParamsAs1DForOutWhenUnconnected=off
  theta : Outport  Port=5  VectorParamsAs1DForOutWhenUnconnected=off
  psi : Outport  Port=6  VectorParamsAs1DForOutWhenUnconnected=off
  wires:
  v_x/1 -> Position Kinematic Model/1(v_x)
  v_y/1 -> Position Kinematic Model/2(v_y)
  r/1 -> Attitude Kinematic Model/3(r)
  p/1 -> Attitude Kinematic Model/1(p)
  v_z/1 -> Position Kinematic Model/3(v_z)
  Position Kinematic Model/1(x) -> x/1
  Position Kinematic Model/2(y) -> y/1
  q/1 -> Attitude Kinematic Model/2(q)
  Position Kinematic Model/3(z) -> z/1
  Attitude Kinematic Model/2(theta) -> theta/1
  Attitude Kinematic Model/1(phi) -> phi/1
  Attitude Kinematic Model/3(psi) -> psi/1

== system quad_with_controller/force mapping/Euler To DCM ==
  euler : Inport
  Demux : Demux  Outputs=3
  MATLAB Function : MATLAB Function  TreatAsAtomicUnit=on
  R : Outport
  wires:
  euler/1 -> Demux/1
  MATLAB Function/1(R) -> R/1
  Demux/1 -> MATLAB Function/3(phi)
  Demux/2 -> MATLAB Function/2(theta)
  Demux/3 -> MATLAB Function/1(psi)

== system quad_with_controller/force_sp mapping/Euler To DCM ==
  euler : Inport
  Demux : Demux  Outputs=3
  MATLAB Function : MATLAB Function  TreatAsAtomicUnit=on
  R : Outport
  wires:
  euler/1 -> Demux/1
  MATLAB Function/1(R) -> R/1
  Demux/1 -> MATLAB Function/3(phi)
  Demux/2 -> MATLAB Function/2(theta)
  Demux/3 -> MATLAB Function/1(psi)

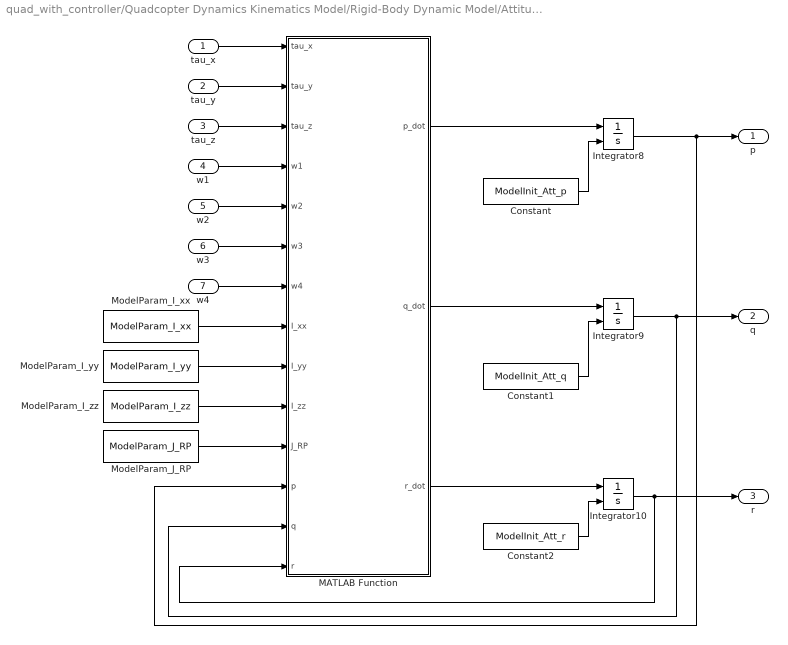
== system quad_with_controller/Quadcopter Dynamics Kinematics Model/Rigid-Body Dynamic Model/Attitude Dynamic Model ==
  tau_x : Inport
  tau_y : Inport  Port=2
  tau_z : Inport  Port=3
  w1 : Inport  Port=4
  w2 : Inport  Port=5
  w3 : Inport  Port=6
  w4 : Inport  Port=7
  Constant : Constant  Value=ModelInit_Att_p
  Constant1 : Constant  Value=ModelInit_Att_q
  Constant2 : Constant  Value=ModelInit_Att_r
  Integrator10 : Integrator  InitialConditionSource=external
  Integrator8 : Integrator  InitialConditionSource=external
  Integrator9 : Integrator  InitialConditionSource=external
  MATLAB Function : MATLAB Function  TreatAsAtomicUnit=on
  ModelParam_I_xx : Constant  Value=ModelParam_I_xx
  ModelParam_I_yy : Constant  Value=ModelParam_I_yy
  ModelParam_I_zz : Constant  Value=ModelParam_I_zz
  ModelParam_J_RP : Constant  Value=ModelParam_J_RP
  p : Outport  VectorParamsAs1DForOutWhenUnconnected=off
  q : Outport  Port=2  VectorParamsAs1DForOutWhenUnconnected=off
  r : Outport  Port=3  VectorParamsAs1DForOutWhenUnconnected=off
  wires:
  ModelParam_I_xx/1 -> MATLAB Function/8(I_xx)
  tau_z/1 -> MATLAB Function/3(tau_z)
  Integrator10/1 -> r/1, MATLAB Function/14(r)
  ModelParam_J_RP/1 -> MATLAB Function/11(J_RP)
  Integrator9/1 -> q/1, MATLAB Function/13(q)
  ModelParam_I_yy/1 -> MATLAB Function/9(I_yy)
  MATLAB Function/3(r_dot) -> Integrator10/1
  MATLAB Function/1(p_dot) -> Integrator8/1
  Integrator8/1 -> p/1, MATLAB Function/12(p)
  tau_y/1 -> MATLAB Function/2(tau_y)
  MATLAB Function/2(q_dot) -> Integrator9/1
  ModelParam_I_zz/1 -> MATLAB Function/10(I_zz)
  w1/1 -> MATLAB Function/4(w1)
  tau_x/1 -> MATLAB Function/1(tau_x)
  w2/1 -> MATLAB Function/5(w2)
  w3/1 -> MATLAB Function/6(w3)
  w4/1 -> MATLAB Function/7(w4)
  Constant/1 -> Integrator8/2
  Constant1/1 -> Integrator9/2
  Constant2/1 -> Integrator10/2

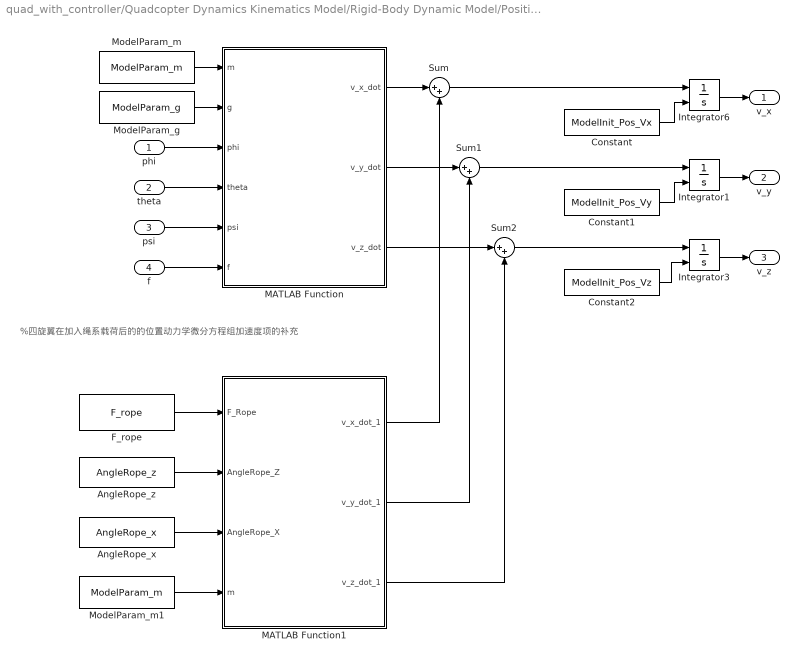
== system quad_with_controller/Quadcopter Dynamics Kinematics Model/Rigid-Body Dynamic Model/Position Dynamic Model ==
  note: %四旋翼在加入绳系载荷后的的位置动力学微分方程组加速度项的补充
  phi : Inport
  theta : Inport  Port=2
  psi : Inport  Port=3
  f : Inport  Port=4
  AngleRope_x : Constant  Value=AngleRope_x
  AngleRope_z : Constant  Value=AngleRope_z
  Constant : Constant  Value=ModelInit_Pos_Vx
  Constant1 : Constant  Value=ModelInit_Pos_Vy
  Constant2 : Constant  Value=ModelInit_Pos_Vz
  F_rope : Constant  Value=F_rope
  Integrator1 : Integrator  InitialConditionSource=external
  Integrator3 : Integrator  InitialConditionSource=external
  Integrator6 : Integrator  InitialConditionSource=external
  MATLAB Function : MATLAB Function  TreatAsAtomicUnit=on
  MATLAB Function1 : MATLAB Function  TreatAsAtomicUnit=on
  ModelParam_g : Constant  Value=ModelParam_g
  ModelParam_m : Constant  Value=ModelParam_m
  ModelParam_m1 : Constant  Value=ModelParam_m
  Sum : Sum  Inputs=|++
  Sum1 : Sum  Inputs=|++
  Sum2 : Sum  Inputs=|++
  v_x : Outport  VectorParamsAs1DForOutWhenUnconnected=off
  v_y : Outport  Port=2  VectorParamsAs1DForOutWhenUnconnected=off
  v_z : Outport  Port=3  VectorParamsAs1DForOutWhenUnconnected=off
  wires:
  ModelParam_g/1 -> MATLAB Function/2(g)
  theta/1 -> MATLAB Function/4(theta)
  ModelParam_m/1 -> MATLAB Function/1(m)
  phi/1 -> MATLAB Function/3(phi)
  f/1 -> MATLAB Function/6(f)
  psi/1 -> MATLAB Function/5(psi)
  Integrator6/1 -> v_x/1
  Integrator1/1 -> v_y/1
  Integrator3/1 -> v_z/1
  F_rope/1 -> MATLAB Function1/1(F_Rope)
  AngleRope_z/1 -> MATLAB Function1/2(AngleRope_Z)
  AngleRope_x/1 -> MATLAB Function1/3(AngleRope_X)
  ModelParam_m1/1 -> MATLAB Function1/4(m)
  MATLAB Function/1(v_x_dot) -> Sum/1
  Sum/1 -> Integrator6/1
  MATLAB Function1/1(v_x_dot_1) -> Sum/2
  MATLAB Function/2(v_y_dot) -> Sum1/1
  Sum1/1 -> Integrator1/1
  MATLAB Function1/2(v_y_dot_1) -> Sum1/2
  MATLAB Function/3(v_z_dot) -> Sum2/1
  Sum2/1 -> Integrator3/1
  MATLAB Function1/3(v_z_dot_1) -> Sum2/2
  Constant/1 -> Integrator6/2
  Constant1/1 -> Integrator1/2
  Constant2/1 -> Integrator3/2

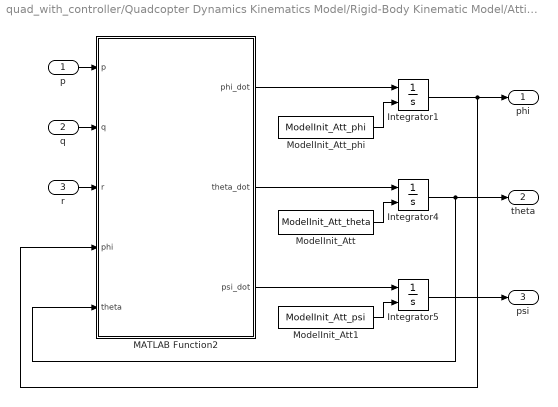
== system quad_with_controller/Quadcopter Dynamics Kinematics Model/Rigid-Body Kinematic Model/Attitude Kinematic Model ==
  p : Inport
  q : Inport  Port=2
  r : Inport  Port=3
  Integrator1 : Integrator  InitialConditionSource=external
  Integrator4 : Integrator  InitialConditionSource=external
  Integrator5 : Integrator  InitialConditionSource=external
  MATLAB Function2 : MATLAB Function  TreatAsAtomicUnit=on
  ModelInit_Att : Constant  Value=ModelInit_Att_theta
  ModelInit_Att1 : Constant  Value=ModelInit_Att_psi
  ModelInit_Att_phi : Constant  Value=ModelInit_Att_phi
  phi : Outport  VectorParamsAs1DForOutWhenUnconnected=off
  theta : Outport  Port=2  VectorParamsAs1DForOutWhenUnconnected=off
  psi : Outport  Port=3  VectorParamsAs1DForOutWhenUnconnected=off
  wires:
  r/1 -> MATLAB Function2/3(r)
  MATLAB Function2/1(phi_dot) -> Integrator1/1
  q/1 -> MATLAB Function2/2(q)
  Integrator1/1 -> MATLAB Function2/4(phi), phi/1
  Integrator4/1 -> theta/1, MATLAB Function2/5(theta)
  Integrator5/1 -> psi/1
  p/1 -> MATLAB Function2/1(p)
  MATLAB Function2/3(psi_dot) -> Integrator5/1
  MATLAB Function2/2(theta_dot) -> Integrator4/1
  ModelInit_Att_phi/1 -> Integrator1/2
  ModelInit_Att/1 -> Integrator4/2
  ModelInit_Att1/1 -> Integrator5/2

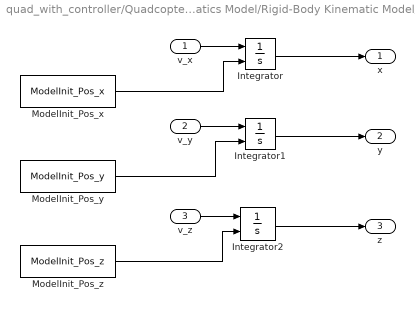
== system quad_with_controller/Quadcopter Dynamics Kinematics Model/Rigid-Body Kinematic Model/Position Kinematic Model ==
  v_x : Inport
  v_y : Inport  Port=2
  v_z : Inport  Port=3
  Integrator : Integrator  InitialConditionSource=external
  Integrator1 : Integrator  InitialConditionSource=external
  Integrator2 : Integrator  InitialConditionSource=external
  ModelInit_Pos_x : Constant  Value=ModelInit_Pos_x
  ModelInit_Pos_y : Constant  Value=ModelInit_Pos_y
  ModelInit_Pos_z : Constant  Value=ModelInit_Pos_z
  x : Outport  VectorParamsAs1DForOutWhenUnconnected=off
  y : Outport  Port=2  VectorParamsAs1DForOutWhenUnconnected=off
  z : Outport  Port=3  VectorParamsAs1DForOutWhenUnconnected=off
  wires:
  v_z/1 -> Integrator2/1
  Integrator1/1 -> y/1
  Integrator/1 -> x/1
  ModelInit_Pos_z/1 -> Integrator2/2
  Integrator2/1 -> z/1
  v_x/1 -> Integrator/1
  v_y/1 -> Integrator1/1
  ModelInit_Pos_y/1 -> Integrator1/2
  ModelInit_Pos_x/1 -> Integrator/2

== matlab function quad_with_controller/Motor Speed control part/MATLAB Function ==
  data: Thrust input; w_trust output; Roll input; Pitch input; Yaw input; C_T input; C_M input; d input; dw_Roll output; dw_Pitch output; dw_Yaw output
function [w_trust,dw_Roll,dw_Pitch,dw_Yaw] = fcn(Thrust,Roll,Pitch,Yaw,C_T,C_M,d)
% 函数描述：
% 1.作用：计算电机在各通道所需的转速
% 2.函数输入：
%   Thrust： 螺旋桨拉力（机体轴）
%   Roll：滚转通道 x轴反扭力矩（机体轴）
%   Pitch, 俯仰通道 y轴反扭力矩（机体轴）
%   Yaw, 偏航通道 z轴反扭力矩（机体轴）
%   C_T, 螺旋桨拉力系数
%   C_M, 螺旋桨转矩系数
%   d, 机体中心和任一电机的距离(m)
% 3.函数输出：
%   w_trust,提供拉力所需的电机转速（rad/s）
%   dw_Roll,滚转所需的电机转速偏量（rad/s）
%   dw_Pitch, 俯仰所需的电机转速偏量（rad/s）
%   dw_Yaw，偏航所需的电机转速偏量（rad/s）
% 4.四旋翼构型为“X”型，螺旋桨序号如下所示：
%            3↓   1↑
%              \ /
%              / \
%            2↑   4↓
% 
%   其中，↑表示螺旋桨逆时针旋转；↓表示螺旋桨顺时针旋转。

w_trust = sqrt(abs(Thrust/4/C_T));
dw_Roll = Roll/(4*sqrt(2))/d/C_T/w_trust;
dw_Pitch = Pitch/(4*sqrt(2))/d/C_T/w_trust;
dw_Yaw = Yaw/8/C_M/w_trust;
end

== matlab function quad_with_controller/Motor Speed control part/MATLAB Function1 ==
  data: w1 output; w2 output; w3 output; w4 output; w_thrust input; dw_roll input; dw_pitch input; dw_yaw input
function [w1,w2,w3,w4] = fcn(w_thrust,dw_roll,dw_pitch,dw_yaw)
% 函数描述：
% 1.作用：电机混合 
% 2.函数输入：
%   w_trust,提供拉力所需的电机转速（rad/s）
%   dw_Roll,滚转所需的电机转速偏量（rad/s）
%   dw_Pitch, 俯仰所需的电机转速偏量（rad/s）
%   dw_Yaw，偏航所需的电机转速偏量（rad/s）
% 3.函数输出：
%   w1, 电机1 的转速（rad/s）
%   w2, 电机2 的转速（rad/s）
%   w3, 电机3 的转速（rad/s）
%   w4，电机4 的转速（rad/s）
% 4.四旋翼构型为“X”型，螺旋桨序号如下所示：
%            3↓   1↑
%              \ /
%              / \
%            2↑   4↓
% 
%   其中，↑表示螺旋桨逆时针旋转；↓表示螺旋桨顺时针旋转

w1 = w_thrust - dw_roll + dw_pitch + dw_yaw;
w2 = w_thrust + dw_roll - dw_pitch + dw_yaw;
w3 = w_thrust + dw_roll + dw_pitch - dw_yaw;
w4 = w_thrust - dw_roll - dw_pitch - dw_yaw;
end

== matlab function quad_with_controller/force_sp mapping/Euler To DCM/MATLAB Function ==
  data: psi input; R output; theta input; phi input
function R = euler_to_rotation_matrix(psi, theta, phi)
    % 转换角度为弧度
    % psi = deg2rad(psi);
    % theta = deg2rad(theta);
    % phi = deg2rad(phi);

    % 绕 z 轴的旋转矩阵
    Rz = [cos(psi), -sin(psi), 0;
          sin(psi),  cos(psi), 0;
          0,         0,        1];

    % 绕 y 轴的旋转矩阵
    Ry = [cos(theta), 0, sin(theta);
          0,          1, 0;
          -sin(theta), 0, cos(theta)];

    % 绕 x 轴的旋转矩阵
    Rx = [1, 0,          0;
          0, cos(phi), -sin(phi);
          0, sin(phi),  cos(phi)];

    % 总旋转矩阵 R
    R = Rz * Ry * Rx;
end

== matlab function quad_with_controller/Quadcopter Dynamics Kinematics Model/Rigid-Body Kinematic Model/Attitude Kinematic Model/MATLAB Function2 ==
  data: p input; phi_dot output; q input; r input; phi input; theta input; theta_dot output; psi_dot output
function [phi_dot, theta_dot, psi_dot] = fcn(p, q, r, phi, theta)
% 函数描述
% 1.作用：本函数为四旋翼的姿态运动学微分方程组，通过四旋翼的机体角速度
%         计算得到四旋翼的姿态角
% 2.函数输入：
%   p：四旋翼x轴角速度（机体轴)(rad/s)
%   q：四旋翼y轴角速度（机体轴)(rad/s)
%   r：四旋翼z轴角速度（机体轴)(rad/s)
%   phi：滚转角(rad)
%   theta：俯仰角(rad)
% 3.函数输出：
%   phi_dot：滚转角速度
%   theta_dot：俯仰角速度
%   psi_dot：偏航角速度
% 4.四旋翼构型为“X”型，螺旋桨序号如下所示：
%            3↓   1↑
%              \ /
%              / \
%            2↑   4↓
%   其中，↑表示螺旋桨逆时针旋转；↓表示螺旋桨顺时针旋转。

phi_dot = p + q * tan(theta) * sin(phi) + r * tan(theta) * cos(phi);
theta_dot = q * cos(phi) - r * sin(phi);
psi_dot = (q * sin(phi) + r * cos(phi)) / cos(theta);
end

== matlab function quad_with_controller/Quadcopter Dynamics Kinematics Model/Control Effectiveness Model/MATLAB Function ==
  data: w1 input; f output; w2 input; w3 input; w4 input; c_T input; c_M input; d input; tau_x output; tau_y output; tau_z output
function [f, tau_x, tau_y, tau_z] = fcn(w1, w2, w3, w4, c_T, c_M, d)
% 函数描述
% 1.作用：本函数用来计算螺旋桨旋转产生的总拉力和反扭力矩。
% 2.函数输入：
%   wi：四个螺旋桨的转速(rad/s)
%   c_T：螺旋桨拉力系数
%   c_M：螺旋桨转矩系数
%   d：机体中心和任一电机的距离(m)
% 3.函数输出：
%   f：螺旋桨拉力（机体轴）
%   tau_x：x轴反扭力矩（机体轴）
%   tau_y：y轴反扭力矩（机体轴）
%   tau_z：z轴反扭力矩（机体轴）
% 4.四旋翼构型为“X”型，螺旋桨序号如下所示：
%            3↓   1↑
%              \ /
%              / \
%            2↑   4↓
%                   
%   其中，↑表示螺旋桨逆时针旋转；↓表示螺旋桨顺时针旋转。

f = c_T * (w1^2 + w2^2 + w3^2 + w4^2);
tau_x = d * c_T * (sqrt(2)/2) * (-w1^2 + w2^2 + w3^2 - w4^2);
tau_y = d * c_T * (sqrt(2)/2) * (w1^2 - w2^2 + w3^2 - w4^2);
tau_z = c_M * (w1^2 + w2^2 - w3^2 - w4^2);
end

== matlab function quad_with_controller/Quadcopter Dynamics Kinematics Model/Rigid-Body Dynamic Model/Position Dynamic Model/MATLAB Function1 ==
  data: F_Rope input; v_x_dot_1 output; AngleRope_Z input; AngleRope_X input; v_y_dot_1 output; v_z_dot_1 output; m input
function [v_x_dot_1, v_y_dot_1, v_z_dot_1] = fcn(F_Rope, AngleRope_Z, AngleRope_X, m)
% 函数描述
% 1.作用：本函数为四旋翼在加入绳系载荷后的的位置动力学微分方程组加速度项的补充;
% 2.函数输入：
%	F_Rope: 货物通过绳索作用给无人机的拉力（N）
%	AngleRope_Z：绳索与OZ_e轴的夹角（rad）
%	AngleRope_X：拉力F_Rope投影在XOY_e平面后与OX_e轴的夹角（rad）
%   m：四旋翼飞行器质量(kg)
% 3.函数输出：
%   v_x_dot_1：地球坐标系下沿x轴的速度的导数补充项
%   v_y_dot_1：地球坐标系下沿y轴的速度的导数补充项
%   v_z_dot_1：地球坐标系下沿z轴的速度的导数补充项
% 4.补充：本函数描述重物通过绳索给无人机施加的力大小方向均已知

v_x_dot_1 = (1/m)*F_Rope*sin(AngleRope_Z)*cos(AngleRope_X);
v_y_dot_1 = (1/m)*F_Rope*sin(AngleRope_Z)*sin(AngleRope_X);
v_z_dot_1 = (1/m)*F_Rope*cos(AngleRope_Z);
end

== matlab function quad_with_controller/Quadcopter Dynamics Kinematics Model/Rigid-Body Dynamic Model/Position Dynamic Model/MATLAB Function ==
  data: m input; g input; phi input; theta input; psi input; f input; v_x_dot output; v_y_dot output; v_z_dot output
function [v_x_dot, v_y_dot, v_z_dot] = fcn(m, g, phi, theta, psi, f)
% 函数描述
% 1.作用：本函数为四旋翼的位置动力学微分方程组，通过四旋翼所受拉力、姿态角
%         计算得到四旋翼飞行器的加速度
% 2.函数输入：
%   m：四旋翼飞行器质量(kg)
%   g：重力加速度(m/s^2)
%   phi：滚转角(rad)
%   theta：俯仰角(rad)
%   psi：偏航角(rad)
%   f：螺旋桨产生的总拉力(N)
% 3.函数输出：
%   v_x_dot：地球坐标系下沿x轴的速度的导数
%   v_y_dot：地球坐标系下沿y轴的速度的导数
%   v_z_dot：地球坐标系下沿z轴的速度的导数
% 4.四旋翼构型为“X”型，螺旋桨序号如下所示：
%            3↓   1↑
%              \ /
%              / \
%            2↑   4↓
%   其中，↑表示螺旋桨逆时针旋转；↓表示螺旋桨顺时针旋转。

v_x_dot = -f * (1/m) * (cos(psi) * sin(theta) * cos(phi) + sin(psi) * sin(phi));
v_y_dot = -f * (1/m) * (sin(psi) * sin(theta) * cos(phi) - cos(psi) * sin(phi));
v_z_dot = g - f * (1/m) * cos(phi) * cos(theta);
end

== matlab function quad_with_controller/Quadcopter Dynamics Kinematics Model/Rigid-Body Dynamic Model/Attitude Dynamic Model/MATLAB Function ==
  data: tau_x input; p_dot output; tau_y input; tau_z input; w1 input; w2 input; w3 input; w4 input; I_xx input; I_yy input; I_zz input; J_RP input; p input; q input; r input; q_dot output; r_dot output
function [p_dot, q_dot, r_dot] = fcn(tau_x, tau_y, tau_z, w1, w2, w3, w4, I_xx, I_yy, I_zz, J_RP, p, q, r)
% 函数描述
% 1.作用：本函数为四旋翼的姿态动力学微分方程组，通过四旋翼所受力矩和螺旋
%         桨转速计算得到四旋翼的机体角速度
% 2.函数输入：
%   wi：四个螺旋桨的转速(rad/s)
%   tau_x：x轴反扭力矩（机体轴）(N·m)
%   tau_y：y轴反扭力矩（机体轴）(N·m)
%   tau_z：z轴反扭力矩（机体轴）(N·m)
%   I_xx：四旋翼x轴转动惯量(kg·m^2)
%   I_yy：四旋翼y轴转动惯量(kg·m^2)
%   I_zz：四旋翼z轴转动惯量(kg·m^2)
%   J_RP：整个电机转子和螺旋桨绕转轴的总转动惯量(kg·m^2)
%   p：四旋翼x轴角速度（机体轴)(rad/s)
%   q：四旋翼y轴角速度（机体轴)(rad/s)
%   r：四旋翼z轴角速度（机体轴)(rad/s)
% 3.函数输出：
%   p_dot：四旋翼x轴角加速度（机体轴)
%   q_dot：四旋翼y轴角加速度（机体轴)
%   r_dot：四旋翼z轴角加速度（机体轴)
% 4.四旋翼构型为“X”型，螺旋桨序号如下所示：
%            3↓   1↑
%              \ /
%              / \
%            2↑   4↓
%   其中，↑表示螺旋桨逆时针旋转；↓表示螺旋桨顺时针旋转。

Omega = -w1 - w2 + w3 + w4;
p_dot = (1/I_xx) * (tau_x + q * r * (I_yy - I_zz) - J_RP * q * Omega);
q_dot = (1/I_yy) * (tau_y + p * r * (I_zz - I_xx) + J_RP * p * Omega);
r_dot = (1/I_zz) * (tau_z + p * q * (I_xx - I_yy) );
end

== matlab function quad_with_controller/force mapping/Euler To DCM/MATLAB Function ==
  data: psi input; R output; theta input; phi input
function R = euler_to_rotation_matrix(psi, theta, phi)
    % 转换角度为弧度
    % psi = deg2rad(psi);
    % theta = deg2rad(theta);
    % phi = deg2rad(phi);

    % 绕 z 轴的旋转矩阵
    Rz = [cos(psi), -sin(psi), 0;
          sin(psi),  cos(psi), 0;
          0,         0,        1];

    % 绕 y 轴的旋转矩阵
    Ry = [cos(theta), 0, sin(theta);
          0,          1, 0;
          -sin(theta), 0, cos(theta)];

    % 绕 x 轴的旋转矩阵
    Rx = [1, 0,          0;
          0, cos(phi), -sin(phi);
          0, sin(phi),  cos(phi)];

    % 总旋转矩阵 R
    R = Rz * Ry * Rx;
end
